simulink model "ergasia4senario1"  (R2019a)
settings: Solver=VariableStepAuto  StartTime=0.0  StopTime=10000  RelTol=1e-3
libraries: commdigbbndpm3 x2, commsink2 x1, commrandsrc3 x1
settings Model: Creator=giannis  LastModifiedBy=giannis

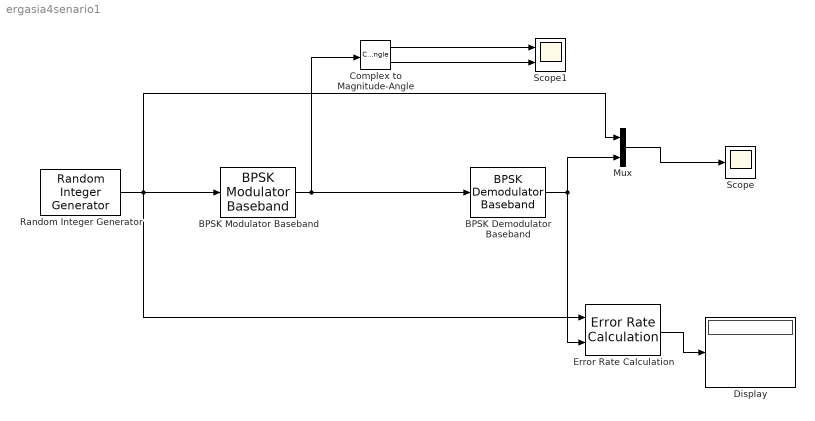
== system ergasia4senario1 ==
  BPSK Demodulator Baseband : commdigbbndpm3/BPSK Demodulator Baseband  DecType=Hard decision  VarSource=Dialog  Variance=1  Ph=0  outDtype=double  derotateFactorWordLen=16  derotateFactorDataTypeStr=Inherit: Same word length as input  derotateFactorLastDataTypeStr=Inherit: Same word length as input
      settings: SourceProductName=Communications Toolbox
  BPSK Modulator Baseband : commdigbbndpm3/BPSK Modulator Baseband  Ph=0  outDtype=double  outWordLen=16  outUDDataType=sfix(16)  outFracLenMode=Best precision  outFracLen=15  outDataTypeStr=double  outLastDataTypeStr=double
      settings: SourceProductName=Communications Toolbox
  Complex to Magnitude-Angle : ComplexToMagnitudeAngle
  Display : Display
  Error Rate Calculation : commsink2/Error Rate Calculation  N=0  st_delay=0  cp_mode=Entire frame  subframe=[]  PMode=Port  WsName=ErrorVec  RsMode2=off  stop=off  numErr=100  maxBits=1e6
      settings: SourceProductName=Communications Toolbox
  Mux : Mux  Inputs=2
  Random Integer Generator : commrandsrc3/Random Integer Generator  SetSize=2  SeedSource=Auto  Seed=0  SampleTime=1  SamplesPerFrame=1  OutputDataType=double  SimulateUsing=Interpreted execution
      settings: SourceProductName=Communications Toolbox
  Scope : Scope
  Scope1 : Scope  NumInputPorts=2
  wires:
  Error Rate Calculation/1 -> Display/1
  Mux/1 -> Scope/1
  BPSK Demodulator Baseband/1 -> Error Rate Calculation/2, Mux/2
  BPSK Modulator Baseband/1 -> Complex to Magnitude-Angle/1, BPSK Demodulator Baseband/1
  Random Integer Generator/1 -> Error Rate Calculation/1, Mux/1, BPSK Modulator Baseband/1
  Complex to Magnitude-Angle/1 -> Scope1/1
  Complex to Magnitude-Angle/2 -> Scope1/2
